simulink model "DDS"  (R2023a)
settings: Solver=VariableStepAuto  StartTime=0.0  StopTime=1  FixedStep=1e-5  RelTol=1e-3
values from neighbouring files (symbols this model uses):
  bhi = fir2(79,f,mi)    [fir2my.m]
libraries: audiofilters x1, dsphdlfiltering2 x1, dsphdlsigops2 x1
settings Model: Creator=31651  LastModifiedBy=31651
settings OptimizationCC: BlockReduction=off  ConditionallyExecuteInputs=off  DefaultParameterBehavior=Inlined
settings DebuggingCC: AlgebraicLoopMsg=error
settings HardwareCC: ProdBitPerPointer=32  ProdBitPerSizeT=32  ProdBitPerPtrDiffT=32  ProdLargestAtomicFloat=None  ProdIntDivRoundTo=Undefined  ProdEndianess=Unspecified  ProdWordSize=32  ProdHWDeviceType=ASIC/FPGA->ASIC/FPGA  TargetBitPerPointer=64  TargetBitPerSizeT=64  TargetBitPerPtrDiffT=64  TargetLongLongMode=on  TargetIntDivRoundTo=Zero  TargetEndianess=LittleEndian  TargetWordSize=64  TargetHWDeviceType=Custom Processor->MATLAB Host Computer  ProdEqTarget=off

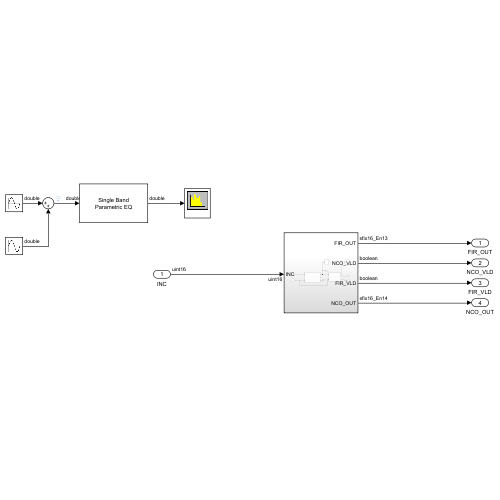
[thumbnail: Simulink's stored preview of the top-level diagram]
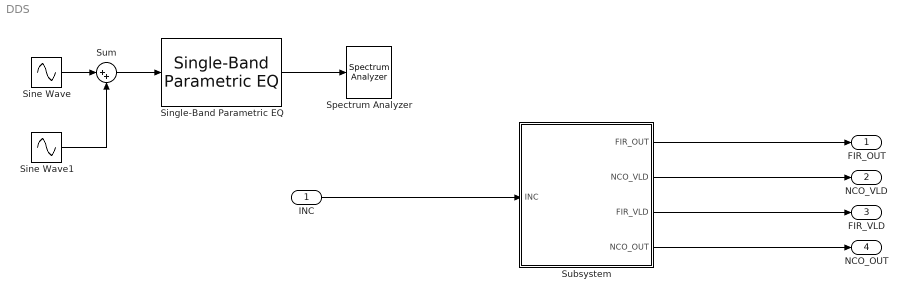
== system DDS ==
  INC : Inport  OutDataTypeStr=uint16
  Sine Wave : Sin  Frequency=1000*2*pi  SampleTime=0
  Sine Wave1 : Sin  Frequency=30000*2*pi  SampleTime=0
  Single-Band Parametric EQ : audiofilters/Single-Band Parametric EQ  FilterOrder=2  Specification=Bandwidth and center frequency  CenterFrequencyPort=off  CenterFrequency=1000.0  BandwidthPort=off  Bandwidth=3000.0  QualityFactorPort=off  QualityFactor=5  PeakGaindBPort=off  PeakGaindB=6.0206  InheritSampleRate=off  SampleRate=44100  SimulateUsing=Code generation
  Spectrum Analyzer : SpectrumAnalyzer  WindowPosition=[811.000000,164.000000,800.000000,500.000000,]  Visible=on  ScopeFrameLocation=window  SampleRateSource=Property  SampleRate=44.1e3  PlotAsTwoSidedSpectrum=off  FrequencyScale=Log  FrequencySpan=Start and stop frequencies  StartFrequency=20  StopFrequency=20e3  YLimits=[-181.87689562,-11.67871519]  ColorLimits=[-20 80]  SelectedToolstripTab=spectrumAnalyzerToolstrip.measurementsTab  DefaultConfigurationName=spbscopes.SpectrumAnalyzerBlockCfg  IsFrequencyInputMode=0  FrequencyVectorPort=0  FrequencyVectorFromPort=0  FrequencyInputRBWPort=0  FrequencyInputRBWFromPort=0
  Subsystem : Subsystem
  Sum : Sum  Inputs=|++
  FIR_OUT : Outport  VectorParamsAs1DForOutWhenUnconnected=off
  NCO_VLD : Outport  Port=2  VectorParamsAs1DForOutWhenUnconnected=off
  FIR_VLD : Outport  Port=3  VectorParamsAs1DForOutWhenUnconnected=off
  NCO_OUT : Outport  Port=4  VectorParamsAs1DForOutWhenUnconnected=off
  wires:
  INC/1 -> Subsystem/1(INC)
  Subsystem/1(FIR_OUT) -> FIR_OUT/1
  Subsystem/2(NCO_VLD) -> NCO_VLD/1
  Subsystem/3(FIR_VLD) -> FIR_VLD/1
  Subsystem/4(NCO_OUT) -> NCO_OUT/1
  Sine Wave/1 -> Sum/1
  Sine Wave1/1 -> Sum/2
  Sum/1 -> Single-Band Parametric EQ/1
  Single-Band Parametric EQ/1 -> Spectrum Analyzer/1

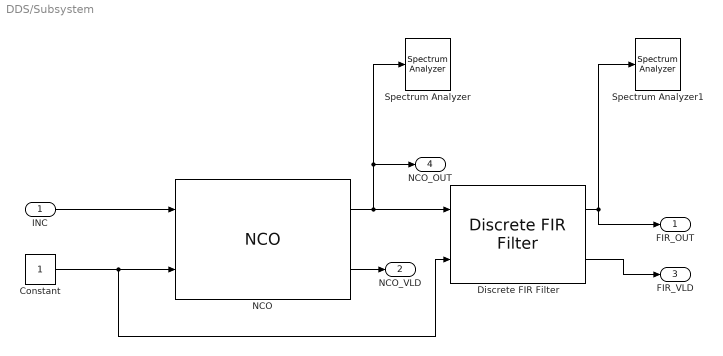
== system DDS/Subsystem ==
  INC : Inport  OutDataTypeStr=uint16
  Constant : Constant  OutDataTypeStr=boolean  SampleTime=1
  Discrete FIR Filter : dsphdlfiltering2/Discrete FIR Filter  NumeratorSource=Property  Numerator=bhi  NumeratorPrototype=[]  FilterStructure=Direct form systolic  SerializationOption=Minimum number of cycles between valid input samples  NumCycles=2  NumberOfMultipliers=2  SimulateUsing=Code generation  roundingMode=Floor  overflowMode=off  CoefficientsDataTypeStr=Inherit: Same word length as input  OutputDataTypeStr=Inherit: Same word length as input  ResetInputPort=off  HDLGlobalReset=off
  NCO : dsphdlsigops2/NCO  PhaseIncrementSource=Input port  PhaseIncrement=6553  PhaseOffsetSource=Property  PhaseOffset=0  DitherSource=Property  NumDitherBits=4  SamplesPerFrame=1  LUTCompress=off  ResetAction=off  Waveform=Sine  PhasePort=off  SimulateUsing=Code generation  AccumulatorWL=16  PhaseQuantization=on  NumQuantizerAccumulatorBits=12  OutputDataType=Binary point scaling  OutputWL=16  OutputFL=14
      settings: LibrarySourceBlock=dsphdlsrcs2/NCO
  Spectrum Analyzer : SpectrumAnalyzer  WindowPosition=[356.000000,292.000000,800.000000,500.000000,]  Visible=on  ScopeFrameLocation=window  Span=50000000  StartFrequency=-25000000  StopFrequency=25000000  YLimits=[-3427.34237515,-2665.71073623]  ColorLimits=[-20 80]  DefaultConfigurationName=spbscopes.SpectrumAnalyzerBlockCfg  IsFrequencyInputMode=0  FrequencyVectorPort=0  FrequencyVectorFromPort=0  FrequencyInputRBWPort=0  FrequencyInputRBWFromPort=0
  Spectrum Analyzer1 : SpectrumAnalyzer  WindowPosition=[1066.000000,273.000000,800.000000,500.000000,]  Visible=on  ScopeFrameLocation=window  Span=50000000  StartFrequency=-25000000  StopFrequency=25000000  YLimits=[-3427.34237515,-2665.71073623]  ColorLimits=[-20 80]  DefaultConfigurationName=spbscopes.SpectrumAnalyzerBlockCfg  IsFrequencyInputMode=0  FrequencyVectorPort=0  FrequencyVectorFromPort=0  FrequencyInputRBWPort=0  FrequencyInputRBWFromPort=0
  FIR_OUT : Outport  VectorParamsAs1DForOutWhenUnconnected=off
  NCO_VLD : Outport  Port=2  VectorParamsAs1DForOutWhenUnconnected=off
  FIR_VLD : Outport  Port=3  VectorParamsAs1DForOutWhenUnconnected=off
  NCO_OUT : Outport  Port=4  VectorParamsAs1DForOutWhenUnconnected=off
  wires:
  NCO/1 -> Discrete FIR Filter/1, NCO_OUT/1, Spectrum Analyzer/1
  Discrete FIR Filter/1 -> FIR_OUT/1, Spectrum Analyzer1/1
  Constant/1 -> NCO/2, Discrete FIR Filter/2
  NCO/2 -> NCO_VLD/1
  Discrete FIR Filter/2 -> FIR_VLD/1
  INC/1 -> NCO/1
